simulink model "randament_pompa"  (R2017b)
settings: Solver=VariableStepAuto  StartTime=0.0  StopTime=10.0  RelTol=1e-3
settings Model: Creator=alinvoicu26  LastModifiedBy=alinvoicu26

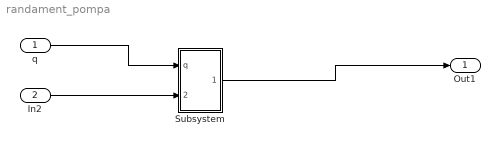
== system randament_pompa ==
  q : Inport
  In2 : Inport  Port=2
  Subsystem : Subsystem
  Out1 : Outport
  wires:
  q/1 -> Subsystem/1(q)
  In2/1 -> Subsystem/2(In2)
  Subsystem/1(Out1) -> Out1/1

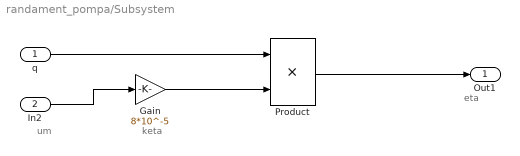
== system randament_pompa/Subsystem ==
  note: eta
  note: keta
  note: um
  q : Inport
  In2 : Inport  Port=2
  Gain : Gain  Gain=8*10^-5
  Product : Product
  Out1 : Outport
  wires:
  Gain/1 -> Product/2
  q/1 -> Product/1
  In2/1 -> Gain/1
  Product/1 -> Out1/1
